simulink library "csu_rrd_rotational_dynamics_lib"  (R2014b)
settings: Solver=ode45  SolverMode=SingleTasking  StartTime=0.0  StopTime=10.0  RelTol=1e-3
libraries: util_common_lib x2, util_info_lib x1
settings Model: ExtModeAutoUpdateStatusClock=off  Creator=daniloviazzo  LastModifiedBy=mstewart

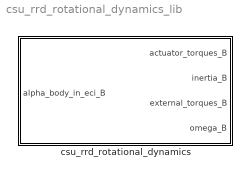
== system csu_rrd_rotational_dynamics_lib ==
  csu_rrd_rotational_dynamics : Subsystem

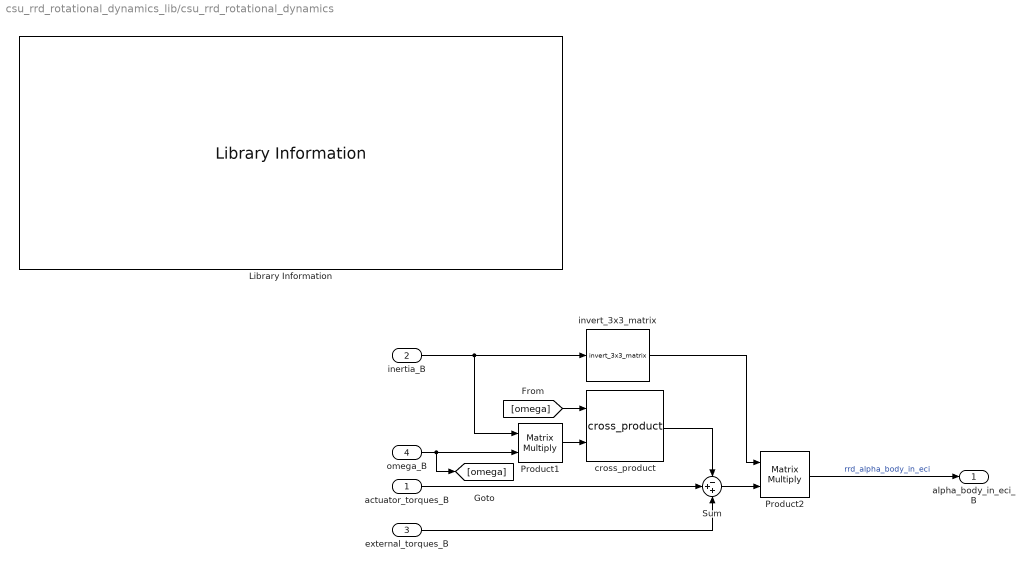
== system csu_rrd_rotational_dynamics_lib/csu_rrd_rotational_dynamics ==
  actuator_torques_B : Inport
  inertia_B : Inport  Port=2
  external_torques_B : Inport  Port=3
  omega_B : Inport  Port=4
  Library Information : util_info_lib/Library Information  owner='NONE'
  Product1 : Product  Multiplication=Matrix(*)  RndMeth=Zero
  Product2 : Product  Multiplication=Matrix(*)  RndMeth=Zero
  Sum : Sum  Inputs=-++
  cross_product : util_common_lib/cross_product  SystemSampleTime=-1
  invert_3x3_matrix : util_common_lib/invert_3x3_matrix  SystemSampleTime=-1
  alpha_body_in_eci_B : Outport
  wires:
  Product2/1 -> alpha_body_in_eci_B/1  "rrd_alpha_body_in_eci"
  Sum/1 -> Product2/2
  invert_3x3_matrix/1 -> Product2/1
  external_torques_B/1 -> Sum/3
  actuator_torques_B/1 -> Sum/2
  cross_product/1 -> Sum/1
  omega_B/1 -> Product1/2, [omega]
  inertia_B/1 -> invert_3x3_matrix/1, Product1/1
  Product1/1 -> cross_product/2
  [omega] -> cross_product/1
